simulink model "Nov19_Serial"  (R2019b)
settings: Solver=FixedStepAuto  StartTime=0.0  StopTime=10.0  FixedStep=1E-3  RelTol=1e-3
undefined symbols (not defined in the file): A0, A1, D0, D1, D10, D11, D12, D13, D2, D3, D4, D5, D6, D7, D8, D9, PTA0, PTA1, PTA2, PTB2, PTB23, PTB3, PTB9, PTC16, PTC17, PTC2, PTC3, PTC4, PTD0, PTD1, PTD2, PTD3
libraries: frdmk64flib x21, nucleoutilitieslib x9
settings Model: PacingRate=0.100000  ExtModeTrigDuration=5  Creator=scotts24  LastModifiedBy=scotts24
settings DataIOCC: ReturnWorkspaceOutputs=off
settings OptimizationCC: PassReuseOutputArgsThreshold=0  MaxStackSize=64
settings DebuggingCC: ParameterTunabilityLossMsg=error  ArithmeticOperatorsInVariantConditions=warning
settings HardwareCC: ProdBitPerPointer=32  ProdBitPerSizeT=32  ProdBitPerPtrDiffT=32  ProdLargestAtomicInteger=Long  ProdLargestAtomicFloat=Double  ProdWordSize=32  ProdHWDeviceType=ARM Compatible->ARM Cortex  UseEmbeddedCoderFeatures=off
settings SFSimCC: SimUseLocalCustomCode=off  MATLABDynamicMemAlloc=off  CustomCodeUndefinedFunction=UseInterfaceOnly
settings RTWCC: SystemTargetFile=ert.tlc  HardwareBoard=NXP FRDM-K64F  TLCOptions="-aInlineSetEventsForThisBaseRateFcn=TLC_FALSE -aSuppressMultiTaskScheduler=TLC_FALSE  -aRateBasedStepFcn=0"  TemplateMakefile=ert_default_tmf  GenerateReport=on  RTWUseLocalCustomCode=off  Toolchain=GNU Tools for ARM Embedded Processors  LaunchReport=on
settings CodeAppCC: ForceParamTrailComments=on  OperatorAnnotations=on
settings ERTTargetCC: ERTCustomFileBanners=off  SupportContinuousTime=on  SupportNonInlinedSFcns=on  RemoveResetFunc=off  ModelStepFunctionPrototypeControlCompliant=off

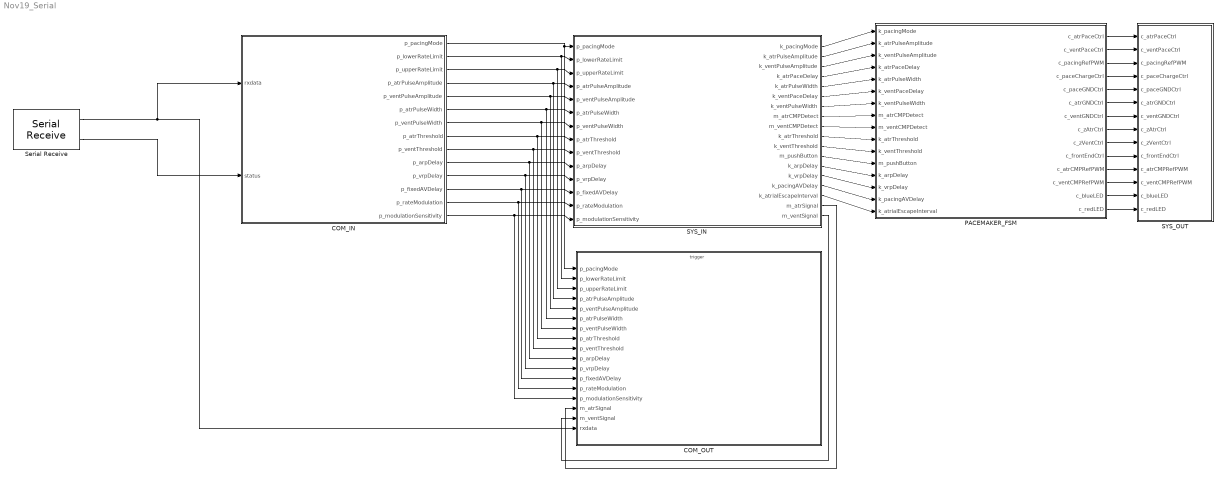
== system Nov19_Serial ==
  COM_IN : Stateflow chart  BlockKeywords=__PRM__SERIALIZED__DATA__:Stateflow Chart,Stateflow Diagram  TreatAsAtomicUnit=on
  COM_OUT : Subsystem  TreatAsAtomicUnit=on
  PACEMAKER_FSM : Stateflow chart  TreatAsAtomicUnit=on
  SYS_IN : Subsystem
  SYS_OUT : Subsystem
  Serial Receive : frdmk64flib/Serial Receive  SCIModule=0  Baudrate=uint32(9600)  Parity=None  StopBits=1  HardwareFlowControl=None  ByteOrder=LittleEndian  DataType=uint8  DataLength=23  BlockingMode=off  OutputStatus=on  SampleTime=-1
      settings: SourceProductName=Simulink Coder Support Package for NXP FRDM-K64F Board
  wires:
  PACEMAKER_FSM/9(c_zVentCtrl) -> SYS_OUT/9(c_zVentCtrl)
  PACEMAKER_FSM/8(c_zAtrCtrl) -> SYS_OUT/8(c_zAtrCtrl)
  PACEMAKER_FSM/7(c_ventGNDCtrl) -> SYS_OUT/7(c_ventGNDCtrl)
  PACEMAKER_FSM/5(c_paceGNDCtrl) -> SYS_OUT/5(c_paceGNDCtrl)
  PACEMAKER_FSM/6(c_atrGNDCtrl) -> SYS_OUT/6(c_atrGNDCtrl)
  PACEMAKER_FSM/4(c_paceChargeCtrl) -> SYS_OUT/4(c_paceChargeCtrl)
  PACEMAKER_FSM/3(c_pacingRefPWM) -> SYS_OUT/3(c_pacingRefPWM)
  PACEMAKER_FSM/2(c_ventPaceCtrl) -> SYS_OUT/2(c_ventPaceCtrl)
  PACEMAKER_FSM/1(c_atrPaceCtrl) -> SYS_OUT/1(c_atrPaceCtrl)
  PACEMAKER_FSM/10(c_frontEndCtrl) -> SYS_OUT/10(c_frontEndCtrl)
  PACEMAKER_FSM/11(c_atrCMPRefPWM) -> SYS_OUT/11(c_atrCMPRefPWM)
  PACEMAKER_FSM/12(c_ventCMPRefPWM) -> SYS_OUT/12(c_ventCMPRefPWM)
  PACEMAKER_FSM/13(c_blueLED) -> SYS_OUT/13(c_blueLED)
  PACEMAKER_FSM/14(c_redLED) -> SYS_OUT/14(c_redLED)
  Serial Receive/1 -> COM_OUT/17(rxdata), COM_IN/1(rxdata)
  Serial Receive/2 -> COM_IN/2(status)
  COM_IN/1(p_pacingMode) -> COM_OUT/1(p_pacingMode), SYS_IN/1(p_pacingMode)
  COM_IN/2(p_lowerRateLimit) -> COM_OUT/2(p_lowerRateLimit), SYS_IN/2(p_lowerRateLimit)
  COM_IN/3(p_upperRateLimit) -> COM_OUT/3(p_upperRateLimit), SYS_IN/3(p_upperRateLimit)
  COM_IN/4(p_atrPulseAmplitude) -> COM_OUT/4(p_atrPulseAmplitude), SYS_IN/4(p_atrPulseAmplitude)
  COM_IN/5(p_ventPulseAmplitude) -> COM_OUT/5(p_ventPulseAmplitude), SYS_IN/5(p_ventPulseAmplitude)
  COM_IN/6(p_atrPulseWidth) -> COM_OUT/6(p_atrPulseWidth), SYS_IN/6(p_atrPulseWidth)
  COM_IN/7(p_ventPulseWidth) -> COM_OUT/7(p_ventPulseWidth), SYS_IN/7(p_ventPulseWidth)
  COM_IN/8(p_atrThreshold) -> COM_OUT/8(p_atrThreshold), SYS_IN/8(p_atrThreshold)
  COM_IN/9(p_ventThreshold) -> COM_OUT/9(p_ventThreshold), SYS_IN/9(p_ventThreshold)
  COM_IN/10(p_arpDelay) -> COM_OUT/10(p_arpDelay), SYS_IN/10(p_arpDelay)
  COM_IN/11(p_vrpDelay) -> COM_OUT/11(p_vrpDelay), SYS_IN/11(p_vrpDelay)
  COM_IN/12(p_fixedAVDelay) -> COM_OUT/12(p_fixedAVDelay), SYS_IN/12(p_fixedAVDelay)
  COM_IN/13(p_rateModulation) -> COM_OUT/13(p_rateModulation), SYS_IN/13(p_rateModulation)
  COM_IN/14(p_modulationSensitivity) -> COM_OUT/14(p_modulationSensitivity), SYS_IN/14(p_modulationSensitivity)
  SYS_IN/1(k_pacingMode) -> PACEMAKER_FSM/1(k_pacingMode)
  SYS_IN/2(k_atrPulseAmplitude) -> PACEMAKER_FSM/2(k_atrPulseAmplitude)
  SYS_IN/3(k_ventPulseAmplitude) -> PACEMAKER_FSM/3(k_ventPulseAmplitude)
  SYS_IN/4(k_atrPaceDelay) -> PACEMAKER_FSM/4(k_atrPaceDelay)
  SYS_IN/5(k_atrPulseWidth) -> PACEMAKER_FSM/5(k_atrPulseWidth)
  SYS_IN/6(k_ventPaceDelay) -> PACEMAKER_FSM/6(k_ventPaceDelay)
  SYS_IN/7(k_ventPulseWidth) -> PACEMAKER_FSM/7(k_ventPulseWidth)
  SYS_IN/8(m_atrCMPDetect) -> PACEMAKER_FSM/8(m_atrCMPDetect)
  SYS_IN/9(m_ventCMPDetect) -> PACEMAKER_FSM/9(m_ventCMPDetect)
  SYS_IN/10(k_atrThreshold) -> PACEMAKER_FSM/10(k_atrThreshold)
  SYS_IN/11(k_ventThreshold) -> PACEMAKER_FSM/11(k_ventThreshold)
  SYS_IN/12(m_pushButton) -> PACEMAKER_FSM/12(m_pushButton)
  SYS_IN/13(k_arpDelay) -> PACEMAKER_FSM/13(k_arpDelay)
  SYS_IN/14(k_vrpDelay) -> PACEMAKER_FSM/14(k_vrpDelay)
  SYS_IN/15(k_pacingAVDelay) -> PACEMAKER_FSM/15(k_pacingAVDelay)
  SYS_IN/16(k_atrialEscapeInterval) -> PACEMAKER_FSM/16(k_atrialEscapeInterval)
  SYS_IN/17(m_atrSignal) -> COM_OUT/15(m_atrSignal)
  SYS_IN/18(m_ventSignal) -> COM_OUT/16(m_ventSignal)

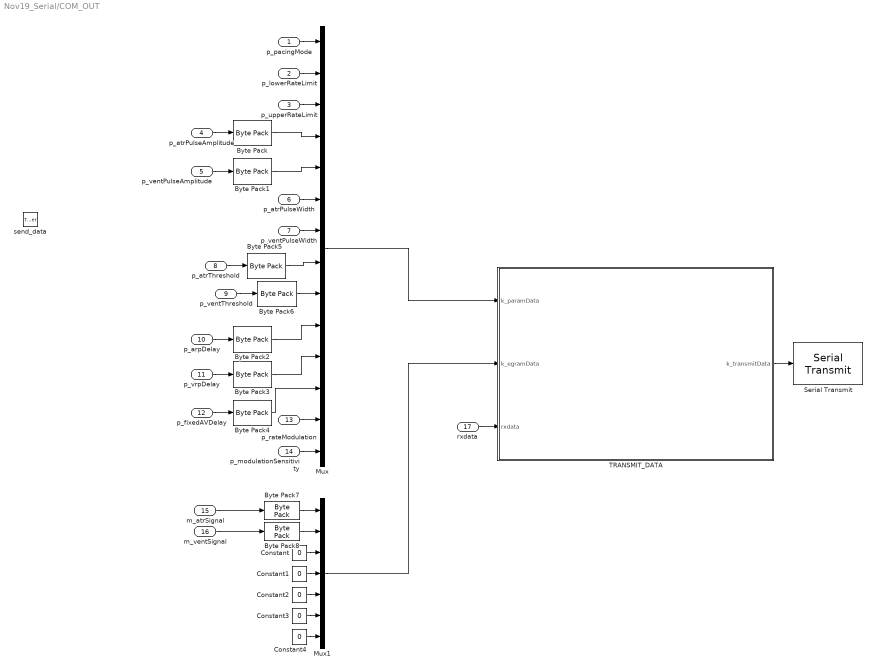
== system Nov19_Serial/COM_OUT ==
  p_pacingMode : Inport
  p_lowerRateLimit : Inport  Port=2
  p_upperRateLimit : Inport  Port=3
  p_atrPulseAmplitude : Inport  Port=4
  p_ventPulseAmplitude : Inport  Port=5
  p_atrPulseWidth : Inport  Port=6
  p_ventPulseWidth : Inport  Port=7
  p_atrThreshold : Inport  Port=8
  p_ventThreshold : Inport  Port=9
  p_arpDelay : Inport  Port=10
  p_vrpDelay : Inport  Port=11
  p_fixedAVDelay : Inport  Port=12
  p_rateModulation : Inport  Port=13
  p_modulationSensitivity : Inport  Port=14
  m_atrSignal : Inport  Port=15
  m_ventSignal : Inport  Port=16
  rxdata : Inport  Port=17
  send_data : TriggerPort  TriggerType=function-call  IsSimulinkFunction=on  FunctionName=send_data  VariantControl=Variant
  Byte Pack{,1..6} (7 alike) : nucleoutilitieslib/Byte Pack  datatypes={'uint16'}  byteAlign=1  blockPlatform=nucleo
      settings: SourceProductName=Embedded Coder Support Package for ARM Cortex-A Processors  SourceProductBaseCode=ECCORTEXA
  Byte Pack7 : nucleoutilitieslib/Byte Pack  datatypes={'double'}  byteAlign=1  blockPlatform=nucleo
      settings: SourceProductName=Embedded Coder Support Package for ARM Cortex-A Processors  SourceProductBaseCode=ECCORTEXA
  Byte Pack8 : nucleoutilitieslib/Byte Pack  datatypes={'double'}  byteAlign=1  blockPlatform=nucleo
      settings: SourceProductName=Embedded Coder Support Package for ARM Cortex-A Processors  SourceProductBaseCode=ECCORTEXA
  Constant{,1..4} (5 alike) : Constant  Value=0  OutDataTypeStr=uint8
  Mux : Mux  Inputs=14
  Mux1 : Mux  Inputs=7
  Serial Transmit : frdmk64flib/Serial Transmit  SCIModule=0  Baudrate=uint32(9600)  Parity=None  StopBits=1  HardwareFlowControl=None  ByteOrder=LittleEndian  BlockingMode=on  OutputStatus=off
      settings: SourceProductName=Simulink Coder Support Package for NXP FRDM-K64F Board
  TRANSMIT_DATA : Stateflow chart  BlockKeywords=__PRM__SERIALIZED__DATA__:Stateflow Chart,Stateflow Diagram  TreatAsAtomicUnit=on
  wires:
  Byte Pack2/1 -> Mux/10
  p_rateModulation/1 -> Mux/13
  p_modulationSensitivity/1 -> Mux/14
  Byte Pack3/1 -> Mux/11
  Byte Pack4/1 -> Mux/12
  p_arpDelay/1 -> Byte Pack2/1
  p_upperRateLimit/1 -> Mux/3
  p_vrpDelay/1 -> Byte Pack3/1
  p_atrPulseAmplitude/1 -> Byte Pack/1
  p_fixedAVDelay/1 -> Byte Pack4/1
  p_ventPulseWidth/1 -> Mux/7
  p_atrPulseWidth/1 -> Mux/6
  Byte Pack1/1 -> Mux/5
  p_ventPulseAmplitude/1 -> Byte Pack1/1
  Byte Pack/1 -> Mux/4
  p_pacingMode/1 -> Mux/1
  p_lowerRateLimit/1 -> Mux/2
  p_atrThreshold/1 -> Byte Pack5/1
  Byte Pack5/1 -> Mux/8
  p_ventThreshold/1 -> Byte Pack6/1
  Byte Pack6/1 -> Mux/9
  Byte Pack7/1 -> Mux1/1
  m_atrSignal/1 -> Byte Pack7/1
  m_ventSignal/1 -> Byte Pack8/1
  Byte Pack8/1 -> Mux1/2
  Mux1/1 -> TRANSMIT_DATA/2(k_egramData)
  Mux/1 -> TRANSMIT_DATA/1(k_paramData)
  rxdata/1 -> TRANSMIT_DATA/3(rxdata)
  TRANSMIT_DATA/1(k_transmitData) -> Serial Transmit/1
  Constant/1 -> Mux1/3
  Constant1/1 -> Mux1/4
  Constant2/1 -> Mux1/5
  Constant3/1 -> Mux1/6
  Constant4/1 -> Mux1/7

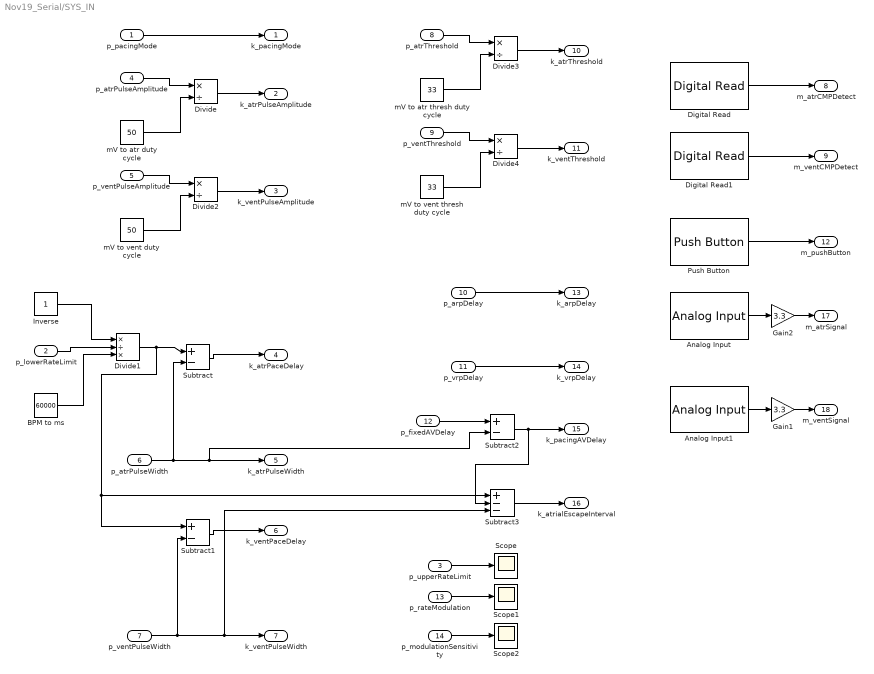
== system Nov19_Serial/SYS_IN ==
  p_pacingMode : Inport
  p_lowerRateLimit : Inport  Port=2
  p_upperRateLimit : Inport  Port=3
  p_atrPulseAmplitude : Inport  Port=4
  p_ventPulseAmplitude : Inport  Port=5
  p_atrPulseWidth : Inport  Port=6
  p_ventPulseWidth : Inport  Port=7
  p_atrThreshold : Inport  Port=8
  p_ventThreshold : Inport  Port=9
  p_arpDelay : Inport  Port=10
  p_vrpDelay : Inport  Port=11
  p_fixedAVDelay : Inport  Port=12
  p_rateModulation : Inport  Port=13
  p_modulationSensitivity : Inport  Port=14
  Analog Input : frdmk64flib/Analog Input  Whichpin=PTB2 (A0)  SampleTime=-1
      settings: SourceProductName=Simulink Coder Support Package for NXP FRDM-K64F Board
  Analog Input1 : frdmk64flib/Analog Input  Whichpin=PTB3 (A1)  SampleTime=-1
      settings: SourceProductName=Simulink Coder Support Package for NXP FRDM-K64F Board
  BPM to ms : Constant  Value=60000
  Digital Read : frdmk64flib/Digital Read  Whichpin=PTC16 (D0)  SampleTime=-1
      settings: SourceProductName=Simulink Coder Support Package for NXP FRDM-K64F Board
  Digital Read1 : frdmk64flib/Digital Read  Whichpin=PTC17 (D1)  SampleTime=-1
      settings: SourceProductName=Simulink Coder Support Package for NXP FRDM-K64F Board
  Divide{,2..4} (4 alike) : Product  Inputs=*/  OutDataTypeStr=uint8
  Divide1 : Product  Inputs=*/*  OutDataTypeStr=double
  Gain1 : Gain  Gain=3.3
  Gain2 : Gain  Gain=3.3
  Inverse : Constant
  Push Button : frdmk64flib/Push Button  Whichswitch=SW2  SampleTime1=-1
      settings: SourceProductName=Simulink Coder Support Package for NXP FRDM-K64F Board
  Scope : Scope
  Scope1 : Scope
  Scope2 : Scope
  Subtract : Sum  Inputs=+-  OutDataTypeStr=uint16
  Subtract1 : Sum  Inputs=+-  OutDataTypeStr=uint16
  Subtract2 : Sum  Inputs=+-  OutDataTypeStr=uint16
  Subtract3 : Sum  Inputs=+--  OutDataTypeStr=uint16
  mV to atr duty cycle : Constant  Value=50
  mV to atr thresh duty cycle : Constant  Value=33
  mV to vent duty cycle : Constant  Value=50
  mV to vent thresh duty cycle : Constant  Value=33
  k_pacingMode : Outport  VectorParamsAs1DForOutWhenUnconnected=off
  k_atrPulseAmplitude : Outport  Port=2  VectorParamsAs1DForOutWhenUnconnected=off
  k_ventPulseAmplitude : Outport  Port=3  VectorParamsAs1DForOutWhenUnconnected=off
  k_atrPaceDelay : Outport  Port=4  VectorParamsAs1DForOutWhenUnconnected=off
  k_atrPulseWidth : Outport  Port=5  VectorParamsAs1DForOutWhenUnconnected=off
  k_ventPaceDelay : Outport  Port=6  VectorParamsAs1DForOutWhenUnconnected=off
  k_ventPulseWidth : Outport  Port=7  VectorParamsAs1DForOutWhenUnconnected=off
  m_atrCMPDetect : Outport  Port=8
  m_ventCMPDetect : Outport  Port=9
  k_atrThreshold : Outport  Port=10  VectorParamsAs1DForOutWhenUnconnected=off
  k_ventThreshold : Outport  Port=11  VectorParamsAs1DForOutWhenUnconnected=off
  m_pushButton : Outport  Port=12
  k_arpDelay : Outport  Port=13  VectorParamsAs1DForOutWhenUnconnected=off
  k_vrpDelay : Outport  Port=14  VectorParamsAs1DForOutWhenUnconnected=off
  k_pacingAVDelay : Outport  Port=15  VectorParamsAs1DForOutWhenUnconnected=off
  k_atrialEscapeInterval : Outport  Port=16  VectorParamsAs1DForOutWhenUnconnected=off
  m_atrSignal : Outport  Port=17
  m_ventSignal : Outport  Port=18
  wires:
  p_atrPulseAmplitude/1 -> Divide/1
  mV to atr duty cycle/1 -> Divide/2
  Divide/1 -> k_atrPulseAmplitude/1
  Subtract/1 -> k_atrPaceDelay/1
  mV to vent duty cycle/1 -> Divide2/2
  p_ventPulseAmplitude/1 -> Divide2/1
  Divide2/1 -> k_ventPulseAmplitude/1
  p_atrPulseWidth/1 -> Subtract/2, Subtract2/2, k_atrPulseWidth/1
  p_ventPulseWidth/1 -> Subtract1/2, Subtract3/3, k_ventPulseWidth/1
  Subtract1/1 -> k_ventPaceDelay/1
  Divide1/1 -> Subtract1/1, Subtract3/1, Subtract/1
  BPM to ms/1 -> Divide1/3
  Inverse/1 -> Divide1/1
  Subtract2/1 -> Subtract3/2, k_pacingAVDelay/1
  Subtract3/1 -> k_atrialEscapeInterval/1
  p_pacingMode/1 -> k_pacingMode/1
  Digital Read/1 -> m_atrCMPDetect/1
  Digital Read1/1 -> m_ventCMPDetect/1
  p_arpDelay/1 -> k_arpDelay/1
  p_vrpDelay/1 -> k_vrpDelay/1
  p_lowerRateLimit/1 -> Divide1/2
  mV to atr thresh duty cycle/1 -> Divide3/2
  p_atrThreshold/1 -> Divide3/1
  Divide3/1 -> k_atrThreshold/1
  p_ventThreshold/1 -> Divide4/1
  mV to vent thresh duty cycle/1 -> Divide4/2
  Divide4/1 -> k_ventThreshold/1
  Push Button/1 -> m_pushButton/1
  p_fixedAVDelay/1 -> Subtract2/1
  p_upperRateLimit/1 -> Scope/1
  p_rateModulation/1 -> Scope1/1
  p_modulationSensitivity/1 -> Scope2/1
  Analog Input/1 -> Gain2/1
  Analog Input1/1 -> Gain1/1
  Gain1/1 -> m_ventSignal/1
  Gain2/1 -> m_atrSignal/1

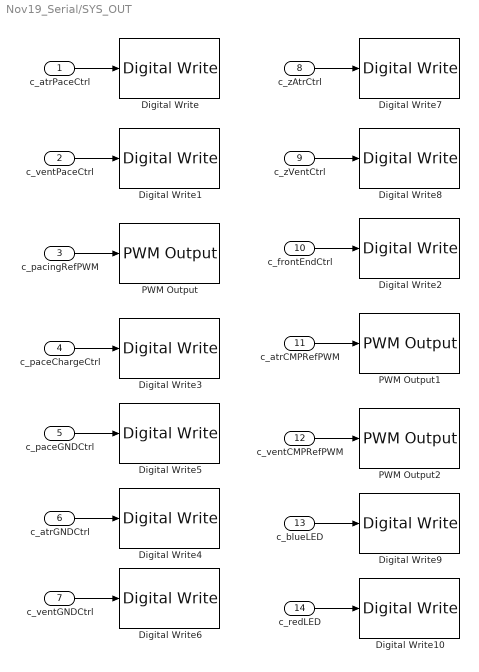
== system Nov19_Serial/SYS_OUT ==
  c_atrPaceCtrl : Inport
  c_ventPaceCtrl : Inport  Port=2
  c_pacingRefPWM : Inport  Port=3
  c_paceChargeCtrl : Inport  Port=4
  c_paceGNDCtrl : Inport  Port=5
  c_atrGNDCtrl : Inport  Port=6
  c_ventGNDCtrl : Inport  Port=7
  c_zAtrCtrl : Inport  Port=8
  c_zVentCtrl : Inport  Port=9
  c_frontEndCtrl : Inport  Port=10
  c_atrCMPRefPWM : Inport  Port=11
  c_ventCMPRefPWM : Inport  Port=12
  c_blueLED : Inport  Port=13
  c_redLED : Inport  Port=14
  Digital Write : frdmk64flib/Digital Write  Whichpin=PTA0 (D8)
      settings: SourceProductName=Simulink Coder Support Package for NXP FRDM-K64F Board
  Digital Write1 : frdmk64flib/Digital Write  Whichpin=PTC4 (D9)
      settings: SourceProductName=Simulink Coder Support Package for NXP FRDM-K64F Board
  Digital Write10 : frdmk64flib/Digital Write  Whichpin=RED_LED
      settings: SourceProductName=Simulink Coder Support Package for NXP FRDM-K64F Board
  Digital Write2 : frdmk64flib/Digital Write  Whichpin=PTD1 (D13)
      settings: SourceProductName=Simulink Coder Support Package for NXP FRDM-K64F Board
  Digital Write3 : frdmk64flib/Digital Write  Whichpin=PTB9 (D2)
      settings: SourceProductName=Simulink Coder Support Package for NXP FRDM-K64F Board
  Digital Write4 : frdmk64flib/Digital Write  Whichpin=PTD2 (D11)
      settings: SourceProductName=Simulink Coder Support Package for NXP FRDM-K64F Board
  Digital Write5 : frdmk64flib/Digital Write  Whichpin=PTD0 (D10)
      settings: SourceProductName=Simulink Coder Support Package for NXP FRDM-K64F Board
  Digital Write6 : frdmk64flib/Digital Write  Whichpin=PTD3 (D12)
      settings: SourceProductName=Simulink Coder Support Package for NXP FRDM-K64F Board
  Digital Write7 : frdmk64flib/Digital Write  Whichpin=PTB23 (D4)
      settings: SourceProductName=Simulink Coder Support Package for NXP FRDM-K64F Board
  Digital Write8 : frdmk64flib/Digital Write  Whichpin=PTC3 (D7)
      settings: SourceProductName=Simulink Coder Support Package for NXP FRDM-K64F Board
  Digital Write9 : frdmk64flib/Digital Write  Whichpin=BLUE_LED
      settings: SourceProductName=Simulink Coder Support Package for NXP FRDM-K64F Board
  PWM Output : frdmk64flib/PWM Output  Whichpin=PTA2 (D5)  InitialFrequency=2000  InitialDutyCycle=0
      settings: SourceProductName=Simulink Coder Support Package for NXP FRDM-K64F Board
  PWM Output1 : frdmk64flib/PWM Output  Whichpin=PTC2 (D6)  InitialFrequency=2000  InitialDutyCycle=0
      settings: SourceProductName=Simulink Coder Support Package for NXP FRDM-K64F Board
  PWM Output2 : frdmk64flib/PWM Output  Whichpin=PTA1 (D3)  InitialFrequency=2000  InitialDutyCycle=0
      settings: SourceProductName=Simulink Coder Support Package for NXP FRDM-K64F Board
  wires:
  c_atrPaceCtrl/1 -> Digital Write/1
  c_ventPaceCtrl/1 -> Digital Write1/1
  c_pacingRefPWM/1 -> PWM Output/1
  c_paceChargeCtrl/1 -> Digital Write3/1
  c_atrGNDCtrl/1 -> Digital Write4/1
  c_paceGNDCtrl/1 -> Digital Write5/1
  c_ventGNDCtrl/1 -> Digital Write6/1
  c_zAtrCtrl/1 -> Digital Write7/1
  c_zVentCtrl/1 -> Digital Write8/1
  c_frontEndCtrl/1 -> Digital Write2/1
  c_atrCMPRefPWM/1 -> PWM Output1/1
  c_ventCMPRefPWM/1 -> PWM Output2/1
  c_redLED/1 -> Digital Write10/1
  c_blueLED/1 -> Digital Write9/1

== stateflow chart Nov19_Serial/COM_IN ==
  settings: executeAtInitialization=1
  state SET_PARAM
    entry:
    p_pacingMode = rxdata(3);
    p_lowerRateLimit = rxdata(4);
    p_upperRateLimit = rxdata(5);
    p_atrPulseAmplitude = typecast(rxdata(6:7), 'uint16');
    p_ventPulseAmplitude = typecast(rxdata(8:9), 'uint16');
    p_atrPulseWidth = rxdata(10);
    p_ventPulseWidth = rxdata(11);
    p_atrThreshold = typecast(rxdata(12:13), 'uint16');
    p_ventThreshold = typecast(rxdata(14:15), 'uint16');
    p_arpDelay = typecast(rxdata(16:17), 'uint16');
    p_vrpDelay = typecast(rxdata(18:19), 'uint16');
    p_fixedAVDelay = typecast(rxdata(20:21), 'uint16');
    p_rateModulation = rxdata(22);
    p_modulationSensitivity = rxdata(23);
  state INIT
    %setting default values for the programmable parameters
    entry:
    p_pacingMode = 0;
    p_lowerRateLimit = 60;
    p_upperRateLimit = 120;
    p_atrPulseAmplitude = 3500;
    p_ventPulseAmplitude = 3500;
    p_atrPulseWidth = 10;
    p_ventPulseWidth = 10;
    p_atrThreshold = 2640;
    p_ventThreshold = 2640;
    p_arpDelay = 250;
    p_vrpDelay = 320;
    p_fixedAVDelay = 150;
    p_rateModulation = 0;
    p_modulationSensitivity = 8;
    k_sampleRate = 10;
  state STANDBY
    %waiting for COM
  state ECHO_PARAM
    entry:
    send_data();
  state ECHO_EGRAM
    entry:
    send_data();
  SET_PARAM -> STANDBY
  (default) -> INIT
  (junction 40) -> SET_PARAM [order 2] : [rxdata(2) == hex2dec('55')]
  INIT -> STANDBY
  STANDBY -> (junction 40) : [status == 0 && rxdata(1) == hex2dec('16')]
  (junction 40) -> ECHO_PARAM [order 1] : [rxdata(2) == hex2dec('22')]
  (junction 40) -> ECHO_EGRAM [order 3] : [rxdata(2) == hex2dec('47')]
  ECHO_EGRAM -> STANDBY [order 1] : [rxdata(2) == hex2dec('62')]
  ECHO_PARAM -> STANDBY
  ECHO_EGRAM -> ECHO_EGRAM [order 2] : [after(k_sampleRate, msec)]
  data: rxdata input uint8; status input uint8; p_pacingMode output uint8; p_lowerRateLimit output uint8; p_upperRateLimit output uint8; p_atrPulseAmplitude output uint16; p_ventPulseAmplitude output uint16; p_atrPulseWidth output uint8; p_ventPulseWidth output uint8; p_atrThreshold output uint16; p_ventThreshold output uint16; p_arpDelay output uint16; p_vrpDelay output uint16; p_fixedAVDelay output uint16; p_rateModulation output uint8; p_modulationSensitivity output uint8; k_sampleRate local uint8

== stateflow chart Nov19_Serial/COM_OUT/TRANSMIT_DATA ==
  state TRANSMIT_PARAMS
    k_transmitData = k_paramData;
  state INIT
  state TRANSMIT_EGRAM
    k_transmitData = k_egramData;
  INIT -> TRANSMIT_PARAMS [order 1] : [rxdata(2) == hex2dec('22')]
  (default) -> INIT
  INIT -> TRANSMIT_EGRAM [order 2] : [rxdata(2) == hex2dec('47')]
  data: k_paramData input uint8; k_egramData input uint8; rxdata input uint8; k_transmitData output uint8

== stateflow chart Nov19_Serial/PACEMAKER_FSM ==
  note: In this state, we are allowing current to flow from C22
      | across the impendence of the atrium to C21 to generate an
      | artificial pace in the atrium. The LED is set to blue.
  note: In this state, we are allowing current to flow from C22
      | across the impendence of the ventricle to C21 to generate an
      | artificial pace in the ventricle. The LED is set to red.
  state A_PACING
    entry:
    c_paceChargeCtrl = false;
    c_paceGNDCtrl = true;
    c_ventPaceCtrl = false;
    c_ventGNDCtrl = false;
    c_zAtrCtrl = false;
    c_zVentCtrl = false;
    c_atrGNDCtrl = false;
    c_atrPaceCtrl = true;
    c_blueLED = true;
  state V_PACING
    entry:
    c_paceChargeCtrl = false;
    c_paceGNDCtrl = true;
    c_atrPaceCtrl = false;
    c_atrGNDCtrl = false;
    c_zAtrCtrl = false;
    c_zVentCtrl = false;
    c_ventGNDCtrl = false;
    c_ventPaceCtrl = true;
    c_redLED = true;
  note: Move from charging the C22 capacitor to pacing
      | the atrium after the delay atrPaceDelay which is the
      | time in between atrium paces depending on the BPM.
  note: Move from charging the C22 capacitor to pacing
      | the ventricle after the delay ventPaceDelay which is the
      | time in between ventricle paces depending on the BPM.
  note: Move from pacing the ventricle to charging the C22
      | capacitor after the delay ventPulseWidth which is the
      | programmed ventricle pulse width.
  note: Move from pacing the atrium to charging the C22
      | capacitor after the delay atrPulseWidth which is the
      | programmed atrium pulse width.
  state A_CHARGING
    entry:
    c_atrCMPRefPWM = k_atrThreshold;
    c_pacingRefPWM = k_atrPulseAmplitude;
    c_paceGNDCtrl = true;
    c_atrPaceCtrl = false;
    c_zAtrCtrl = false;
    c_zVentCtrl = false;
    c_ventPaceCtrl = false;
    c_ventGNDCtrl = false;
    c_atrGNDCtrl = true;
    c_paceChargeCtrl = true;
    c_blueLED = false;
  state V_CHARGING
    entry:
    c_ventCMPRefPWM = k_ventThreshold;
    c_pacingRefPWM = k_ventPulseAmplitude;
    c_paceGNDCtrl = true;
    c_ventPaceCtrl = false;
    c_zAtrCtrl = false;
    c_zVentCtrl = false;
    c_atrPaceCtrl = false;
    c_atrGNDCtrl = false;
    c_ventGNDCtrl = true;
    c_paceChargeCtrl = true;
    c_redLED = false;
  state INIT
    entry:
    c_frontEndCtrl = true;
    c_pacingRefPWM = 0;
    c_paceChargeCtrl = false;
    c_atrPaceCtrl = false;
    c_ventPaceCtrl = false;
    c_atrGNDCtrl = false;
    c_ventGNDCtrl = false;
    c_paceGNDCtrl = false;
    c_blueLED = false;
    c_redLED = false;
  note: True if the pacing mode is AOO, AAI, or DOO
  note: True if the pacing mode is VOO or VVI
  note: In this state, we are both charging the C22 capacitor,
      | and reversing current flow throug the ventricle in order
      | to create zero net charge. This is done by first
      | ensuring the patient is not directly connected to the
      | voltage supply by setting ventiPaceCtrl to false, which
      | opens the switch to prevent current flow from
      | C22 to C21.
  note: In this state, we are both charging the C22 capacitor,
      | and reversing current flow throug the atrium in order
      | to create zero net charge. This is done by first
      | ensuring the patient is not directly connected to the
      | voltage supply by setting atriPaceCtrl to false, which
      | opens the switch to prevent current flow from
      | C22 to C21.
  note: In this initial state, all switches are open and there is no current
      | flow in the system. The pacemaker then goes to the appropriate
      | atrium or ventricle charging states depending on which mode
      | is being implemented.
  note: This self-loop is used in sensing modes. Sensing does not begin until
      | after the atrium refractory period which is the atrDelay. When
      | a pace is sensed in the atrium, m_atrCMPDetect is set to true
      | and we stay in the charging state because we want to inhibit the next atrium
      | pace. Pushing the button will also satisfy this condition and inhibit a pace.
  note: This self-loop is used in sensing modes. Sensing does not begin until
      | after the ventricle refractory period which is the vtrDelay. When
      | a pace is sensed in the ventricle, m_ventCMPDetect is set to true
      | and we stay in the charging state because we want to inhibit the next ventricle
      | pace. Pushing the button will also satisfy this condition and inhibit a pace.
  V_CHARGING -> A_PACING [order 3] : [after(k_atrialEscapeInterval, msec) && k_pacingMode == 4]
  A_CHARGING -> V_PACING [order 3] : [after(k_pacingAVDelay, msec) && k_pacingMode == 4]
  A_PACING -> A_CHARGING : [after(k_atrPulseWidth, msec)]
  V_PACING -> V_CHARGING : [after(k_ventPulseWidth, msec)]
  A_CHARGING -> A_PACING [order 1] : [after(k_atrPaceDelay, msec)]
  V_CHARGING -> V_PACING [order 1] : [after(k_ventPaceDelay, msec)]
  (default) -> INIT
  INIT -> A_CHARGING [order 2] : [k_pacingMode == 0 || k_pacingMode == 2 || k_pacingMode == 4]
  INIT -> V_CHARGING [order 1] : [k_pacingMode == 1 || k_pacingMode == 3]
  V_CHARGING -> V_CHARGING [order 2] : [after(k_vrpDelay, msec) && k_pacingMode == 3 && m_ventCMPDetect == true || m_pushButton == true]
  A_CHARGING -> A_CHARGING [order 2] : [after(k_arpDelay, msec) && k_pacingMode == 2 && m_atrCMPDetect == true || m_pushButton == true]
  data: c_atrPaceCtrl output boolean; c_ventPaceCtrl output boolean; c_pacingRefPWM output uint8; c_paceChargeCtrl output boolean; c_paceGNDCtrl output boolean; c_atrGNDCtrl output boolean; c_ventGNDCtrl output boolean; c_zAtrCtrl output boolean; c_zVentCtrl output boolean; k_pacingMode input uint8; k_atrPulseAmplitude input uint8; k_ventPulseAmplitude input uint8; k_atrPaceDelay input uint16; k_atrPulseWidth input uint8; k_ventPaceDelay input uint16; k_ventPulseWidth input uint8; m_atrCMPDetect input boolean; m_ventCMPDetect input boolean; c_frontEndCtrl output boolean; c_atrCMPRefPWM output uint8; k_atrThreshold input uint8; k_ventThreshold input uint8; c_ventCMPRefPWM output uint8; m_pushButton input boolean; c_blueLED output boolean; c_redLED output boolean; k_arpDelay input uint16; k_vrpDelay input uint16; k_pacingAVDelay input uint16; k_atrialEscapeInterval input uint16
